simulink model "GS_model"  (R2018b)
settings: Solver=ode5  StartTime=0.0  StopTime=SimuStopTime  FixedStep=T_Simu  RelTol=1e-3
InitFcn:
  | Initial
undefined symbols (not defined in the file or in its folder): Aba10, Aba20, aeroCIP2006_S, aeroCIP2006_X, aeroCIP2006_Y, Agl0, Ass_kS, Ass_n1, Ass_n2, Ass_n3, Ass_n4, Ass_Noise, Ass_R, Ass_Resolution, Ass_TmOrder, AssA_Fix_Abs, AssB_Fix_Abs, AssC_Fix_Abs, AssD_Fix_Abs, AssE_Fix_Aps, AssF_Fix_Aps, C, c_max, c_min, Cd, CenterOfFigNX, CenterOfFigNY, CenterOfFigNZ, CenterOfFigP1, CenterOfFigP2, CenterOfFigPX, CenterOfFigPY, CenterOfFigPZ, Cmu, Crou, DEG2RAD, DiscIntNeverNeededParam, Eg_Dir, Eg_F, Eg_PrepareTime, Eg_r_L_L, Fw_Abf, Fw_Hmax, Fw_J, Fw_Spd0, Fw_Tmax, git_hash_BaseLine, git_hash_Project, Gnss_Noise_Pos, Gnss_Noise_Vel, Gnss_PropgationTime, GyroA_Fix_Abg, GyroA_Noise, GyroB_Fix_Abg, GyroB_Noise, GyroC_Fix_Abg, GyroC_Noise, GyroD_Fix_Abg, GyroD_Noise, h ... (+94)
libraries: simulink x308, sharedutil x46, aerolibutil x37, sharedtransform x31, vrlib x14, aerolibgravity2 x2
(part 11 of 20)

== system GS_model/Subsystem2/Subsystem/Sensor/Ass/BodyAss(A&B&C&D)Model/Subsystem/AssErrModel ==
  AssCur : Inport
  TC_AssGNDSet : Inport  Port=2
  TC_AssErr_Constant : Inport  Port=3
  TC_AssErr_WildValue : Inport  Port=4
  TC_AssErr_Jump : Inport  Port=5
  TC_AssErr_Wave : Inport  Port=6
  AssNum : Inport  Port=7
  AssErrSet : Subsystem
  Constant : Constant  Value=0
  Demux : Demux  Outputs=2
  Demux1 : Demux  Outputs=2
  Demux2 : Demux  Outputs=[1;3]
  Demux3 : Demux  Outputs=[1;2]
  Demux4 : Demux  Outputs=[1;4]
  Demux5 : Demux  Outputs=[1;5]
  If : If  IfExpression=u1 == 1
  If Action Subsystem : Subsystem  TreatAsAtomicUnit=on
  If Action Subsystem1 : Subsystem  TreatAsAtomicUnit=on
  Logical Operator{1..5} (5 alike) : Logic  Operator=OR  AllPortsSameDT=off  OutDataTypeStr=boolean
  Merge : Merge
  Relational Operator{1..10} (10 alike) : RelationalOperator  Operator===  OutDataTypeStr=boolean  RndMeth=Simplest
  Triggered Subsystem1 : Subsystem  TreatAsAtomicUnit=on
      mask Display: disp('AssChoice')
  Triggered Subsystem2 : Subsystem  TreatAsAtomicUnit=on
      mask Display: disp('AssChoice')
  Triggered Subsystem3 : Subsystem  TreatAsAtomicUnit=on
      mask Display: disp('AssChoice')
  Triggered Subsystem4 : Subsystem  TreatAsAtomicUnit=on
      mask Display: disp('AssChoice')
  Triggered Subsystem5 : Subsystem  TreatAsAtomicUnit=on
      mask Display: disp('AssChoice')
  TM_Ass_Cur : Outport
  wires:
  Demux/2 -> Triggered Subsystem1/1(In1)
  Demux/1 -> Relational Operator9/2, Relational Operator2/2
  Demux2/1 -> Relational Operator4/2, Relational Operator7/2
  Demux3/1 -> Relational Operator6/2, Relational Operator5/2
  Demux3/2 -> Triggered Subsystem4/1(In1)
  TC_AssErr_Constant/1 -> Demux/1
  TC_AssErr_Wave/1 -> Demux3/1
  AssCur/1 -> AssErrSet/1(AssCur)
  Triggered Subsystem1/1(Out1) -> AssErrSet/2(TC_AssErr_Constant)
  Triggered Subsystem3/1(Out1) -> AssErrSet/4(TC_AssErr_Jump)
  Triggered Subsystem4/1(Out1) -> AssErrSet/5(TC_StErr_Wave)
  Demux4/1 -> If/1
  If/1 -> If Action Subsystem/Action
  Demux4/2 -> If Action Subsystem/1(In1)
  If/2 -> If Action Subsystem1/Action
  AssErrSet/1(TM_Ass_Cur) -> If Action Subsystem1/1(In1)
  If Action Subsystem/1(Out1) -> Merge/1
  If Action Subsystem1/1(Out1) -> Merge/2
  Merge/1 -> TM_Ass_Cur/1
  Demux2/2 -> Triggered Subsystem3/1(In1)
  TC_AssErr_Jump/1 -> Demux2/1
  TC_AssErr_WildValue/1 -> Demux1/1
  Demux1/1 -> Relational Operator8/2, Relational Operator3/2
  Demux1/2 -> Triggered Subsystem2/1(In1)
  Triggered Subsystem2/1(Out1) -> AssErrSet/3(TC_AssErr_WildValue)
  TC_AssGNDSet/1 -> Demux5/1
  Demux5/1 -> Relational Operator10/2, Relational Operator1/2
  Demux5/2 -> Triggered Subsystem5/1(In1)
  Triggered Subsystem5/1(Out1) -> Demux4/1
  AssNum/1 -> Relational Operator1/1, Relational Operator2/1, Relational Operator3/1, Relational Operator5/1, Relational Operator4/1
  Relational Operator6/1 -> Logical Operator2/1
  Relational Operator5/1 -> Logical Operator2/2
  Logical Operator2/1 -> Triggered Subsystem4/Enable
  Constant/1 -> Relational Operator10/1, Relational Operator9/1, Relational Operator8/1, Relational Operator7/1, Relational Operator6/1
  Relational Operator7/1 -> Logical Operator1/1
  Relational Operator4/1 -> Logical Operator1/2
  Logical Operator1/1 -> Triggered Subsystem3/Enable
  Relational Operator3/1 -> Logical Operator3/2
  Relational Operator8/1 -> Logical Operator3/1
  Logical Operator3/1 -> Triggered Subsystem2/Enable
  Relational Operator9/1 -> Logical Operator4/1
  Relational Operator2/1 -> Logical Operator4/2
  Logical Operator4/1 -> Triggered Subsystem1/Enable
  Relational Operator10/1 -> Logical Operator5/1
  Relational Operator1/1 -> Logical Operator5/2
  Logical Operator5/1 -> Triggered Subsystem5/Enable

== system GS_model/Subsystem2/Subsystem/Sensor/Ass/BodyAss(A&B&C&D)Model/Subsystem/AssMathModel ==
  note: Sun_s
  Sunshine : Inport
  AbAss : Inport  Port=2
  Sun_b : Inport  Port=3
  kS_Ass : Inport  Port=4
  1/ R_Ass : Gain  Gain=1/Ass_R
  A2mA : Gain  Gain=1000
  AssNoise : RandomNumber  Mean=zeros(4,1)  Variance=(Ass_Noise/3)^2*ones(4,1)  Seed=[1:4]  SampleTime=T_Simu
  Compare To Zero{,1..3} (4 alike) : simulink/Logic and Bit Operations/Compare To Zero  relop=>=  OutDataTypeStr=uint8
  Data Type Conversion{,1..3} (4 alike) : DataTypeConversion  OutDataTypeStr=double
  Dot Product{,1..3} (4 alike) : DotProduct  InputSameDT=on  OutDataTypeStr=Inherit: Inherit via internal rule
  Mux5 : Mux
  Product{,1..2,7} (4 alike) : Product  RndMeth=Zero
  Product{3..6} (4 alike) : Product  Inputs=3  RndMeth=Zero
  Product8 : Product  Multiplication=Matrix(*)  RndMeth=Zero
  Rounding Function : Rounding
  Ss1Face1Normal : Constant  Value=Ass_n1
  Ss1Face2Normal : Constant  Value=Ass_n2
  Ss1Face3Normal : Constant  Value=Ass_n3
  Ss1Face4Normal : Constant  Value=Ass_n4
  Sum1 : Sum  Inputs=++|
  Transpose5 : Math  Operator=transpose  SaturateOnIntegerOverflow=on
  decode : Gain  Gain=Ass_Resolution
  encode : Gain  Gain=1/Ass_Resolution
  mA2A : Gain  Gain=0.001
  AssCur : Outport
  wires:
  Ss1Face1Normal/1 -> Dot Product/2
  Product1/1 -> Mux5/2
  Dot Product/1 -> Product3/2, Compare To Zero/1
  Product7/1 -> Mux5/4
  Dot Product3/1 -> Compare To Zero3/1, Product6/2
  Ss1Face3Normal/1 -> Dot Product2/2
  Ss1Face2Normal/1 -> Dot Product1/2
  Product5/1 -> Product2/2
  kS_Ass/1 -> Product3/3, Product4/3, Product6/3, Product5/3
  Dot Product1/1 -> Compare To Zero1/1, Product4/2
  Product2/1 -> Mux5/3
  Product8/1 -> Dot Product/1, Dot Product1/1, Dot Product2/1, Dot Product3/1
  Transpose5/1 -> Product8/1
  Product/1 -> Mux5/1
  Product6/1 -> Product7/2
  Dot Product2/1 -> Product5/2, Compare To Zero2/1
  Compare To Zero2/1 -> Data Type Conversion2/1
  Data Type Conversion1/1 -> Product4/1
  Sunshine/1 -> Product/1, Product1/1, Product2/1, Product7/1
  Product4/1 -> Product1/2
  Product3/1 -> Product/2
  Ss1Face4Normal/1 -> Dot Product3/2
  Compare To Zero3/1 -> Data Type Conversion3/1
  Compare To Zero/1 -> Data Type Conversion/1
  Data Type Conversion3/1 -> Product6/1
  Data Type Conversion2/1 -> Product5/1
  Data Type Conversion/1 -> Product3/1
  Sun_b/1 -> Product8/2
  AbAss/1 -> Transpose5/1
  Compare To Zero1/1 -> Data Type Conversion1/1
  Mux5/1 -> Sum1/2
  AssNoise/1 -> 1/ R_Ass/1
  1/ R_Ass/1 -> Sum1/1
  mA2A/1 -> AssCur/1
  Sum1/1 -> A2mA/1
  encode/1 -> Rounding Function/1
  Rounding Function/1 -> decode/1
  A2mA/1 -> encode/1
  decode/1 -> mA2A/1

== system GS_model/Subsystem2/Subsystem/Sensor/Ass/BodyAss(A&B&C&D)Model/Subsystem1/AssErrModel ==
  AssCur : Inport
  TC_AssGNDSet : Inport  Port=2
  TC_AssErr_Constant : Inport  Port=3
  TC_AssErr_WildValue : Inport  Port=4
  TC_AssErr_Jump : Inport  Port=5
  TC_AssErr_Wave : Inport  Port=6
  AssNum : Inport  Port=7
  AssErrSet : Subsystem
  Constant : Constant  Value=0
  Demux : Demux  Outputs=2
  Demux1 : Demux  Outputs=2
  Demux2 : Demux  Outputs=[1;3]
  Demux3 : Demux  Outputs=[1;2]
  Demux4 : Demux  Outputs=[1;4]
  Demux5 : Demux  Outputs=[1;5]
  If : If  IfExpression=u1 == 1
  If Action Subsystem : Subsystem  TreatAsAtomicUnit=on
  If Action Subsystem1 : Subsystem  TreatAsAtomicUnit=on
  Logical Operator{1..5} (5 alike) : Logic  Operator=OR  AllPortsSameDT=off  OutDataTypeStr=boolean
  Merge : Merge
  Relational Operator{1..10} (10 alike) : RelationalOperator  Operator===  OutDataTypeStr=boolean  RndMeth=Simplest
  Triggered Subsystem1 : Subsystem  TreatAsAtomicUnit=on
      mask Display: disp('AssChoice')
  Triggered Subsystem2 : Subsystem  TreatAsAtomicUnit=on
      mask Display: disp('AssChoice')
  Triggered Subsystem3 : Subsystem  TreatAsAtomicUnit=on
      mask Display: disp('AssChoice')
  Triggered Subsystem4 : Subsystem  TreatAsAtomicUnit=on
      mask Display: disp('AssChoice')
  Triggered Subsystem5 : Subsystem  TreatAsAtomicUnit=on
      mask Display: disp('AssChoice')
  TM_Ass_Cur : Outport
  wires:
  Logical Operator5/1 -> Triggered Subsystem5/Enable
  Relational Operator1/1 -> Logical Operator5/2
  Relational Operator10/1 -> Logical Operator5/1
  Logical Operator4/1 -> Triggered Subsystem1/Enable
  Relational Operator2/1 -> Logical Operator4/2
  Relational Operator9/1 -> Logical Operator4/1
  Logical Operator3/1 -> Triggered Subsystem2/Enable
  Relational Operator8/1 -> Logical Operator3/1
  Relational Operator3/1 -> Logical Operator3/2
  Logical Operator1/1 -> Triggered Subsystem3/Enable
  Relational Operator4/1 -> Logical Operator1/2
  Relational Operator7/1 -> Logical Operator1/1
  Constant/1 -> Relational Operator6/1, Relational Operator7/1, Relational Operator8/1, Relational Operator9/1, Relational Operator10/1
  Logical Operator2/1 -> Triggered Subsystem4/Enable
  Relational Operator5/1 -> Logical Operator2/2
  Relational Operator6/1 -> Logical Operator2/1
  AssNum/1 -> Relational Operator4/1, Relational Operator5/1, Relational Operator3/1, Relational Operator2/1, Relational Operator1/1
  Triggered Subsystem5/1(Out1) -> Demux4/1
  Demux5/2 -> Triggered Subsystem5/1(In1)
  Demux5/1 -> Relational Operator1/2, Relational Operator10/2
  TC_AssGNDSet/1 -> Demux5/1
  Triggered Subsystem2/1(Out1) -> AssErrSet/3(TC_AssErr_WildValue)
  Demux1/2 -> Triggered Subsystem2/1(In1)
  Demux1/1 -> Relational Operator3/2, Relational Operator8/2
  TC_AssErr_WildValue/1 -> Demux1/1
  TC_AssErr_Jump/1 -> Demux2/1
  Demux2/2 -> Triggered Subsystem3/1(In1)
  Merge/1 -> TM_Ass_Cur/1
  If Action Subsystem1/1(Out1) -> Merge/2
  If Action Subsystem/1(Out1) -> Merge/1
  AssErrSet/1(TM_Ass_Cur) -> If Action Subsystem1/1(In1)
  If/2 -> If Action Subsystem1/Action
  Demux4/2 -> If Action Subsystem/1(In1)
  If/1 -> If Action Subsystem/Action
  Demux4/1 -> If/1
  Triggered Subsystem4/1(Out1) -> AssErrSet/5(TC_StErr_Wave)
  Triggered Subsystem3/1(Out1) -> AssErrSet/4(TC_AssErr_Jump)
  Triggered Subsystem1/1(Out1) -> AssErrSet/2(TC_AssErr_Constant)
  AssCur/1 -> AssErrSet/1(AssCur)
  TC_AssErr_Wave/1 -> Demux3/1
  TC_AssErr_Constant/1 -> Demux/1
  Demux3/2 -> Triggered Subsystem4/1(In1)
  Demux3/1 -> Relational Operator5/2, Relational Operator6/2
  Demux2/1 -> Relational Operator7/2, Relational Operator4/2
  Demux/1 -> Relational Operator2/2, Relational Operator9/2
  Demux/2 -> Triggered Subsystem1/1(In1)

== system GS_model/Subsystem2/Subsystem/Sensor/Ass/BodyAss(A&B&C&D)Model/Subsystem1/AssMathModel ==
  note: Sun_s
  Sunshine : Inport
  AbAss : Inport  Port=2
  Sun_b : Inport  Port=3
  kS_Ass : Inport  Port=4
  1/ R_Ass : Gain  Gain=1/Ass_R
  A2mA : Gain  Gain=1000
  AssNoise : RandomNumber  Mean=zeros(4,1)  Variance=(Ass_Noise/3)^2*ones(4,1)  Seed=[1:4]  SampleTime=T_Simu
  Compare To Zero{,1..3} (4 alike) : simulink/Logic and Bit Operations/Compare To Zero  relop=>=  OutDataTypeStr=uint8
  Data Type Conversion{,1..3} (4 alike) : DataTypeConversion  OutDataTypeStr=double
  Dot Product{,1..3} (4 alike) : DotProduct  InputSameDT=on  OutDataTypeStr=Inherit: Inherit via internal rule
  Mux5 : Mux
  Product{,1..2,7} (4 alike) : Product  RndMeth=Zero
  Product{3..6} (4 alike) : Product  Inputs=3  RndMeth=Zero
  Product8 : Product  Multiplication=Matrix(*)  RndMeth=Zero
  Rounding Function : Rounding
  Ss1Face1Normal : Constant  Value=Ass_n1
  Ss1Face2Normal : Constant  Value=Ass_n2
  Ss1Face3Normal : Constant  Value=Ass_n3
  Ss1Face4Normal : Constant  Value=Ass_n4
  Sum1 : Sum  Inputs=++|
  Transpose5 : Math  Operator=transpose  SaturateOnIntegerOverflow=on
  decode : Gain  Gain=Ass_Resolution
  encode : Gain  Gain=1/Ass_Resolution
  mA2A : Gain  Gain=0.001
  AssCur : Outport
  wires:
  decode/1 -> mA2A/1
  A2mA/1 -> encode/1
  Rounding Function/1 -> decode/1
  encode/1 -> Rounding Function/1
  Sum1/1 -> A2mA/1
  mA2A/1 -> AssCur/1
  1/ R_Ass/1 -> Sum1/1
  AssNoise/1 -> 1/ R_Ass/1
  Mux5/1 -> Sum1/2
  Compare To Zero1/1 -> Data Type Conversion1/1
  AbAss/1 -> Transpose5/1
  Sun_b/1 -> Product8/2
  Data Type Conversion/1 -> Product3/1
  Data Type Conversion2/1 -> Product5/1
  Data Type Conversion3/1 -> Product6/1
  Compare To Zero/1 -> Data Type Conversion/1
  Compare To Zero3/1 -> Data Type Conversion3/1
  Ss1Face4Normal/1 -> Dot Product3/2
  Product3/1 -> Product/2
  Product4/1 -> Product1/2
  Sunshine/1 -> Product7/1, Product2/1, Product1/1, Product/1
  Data Type Conversion1/1 -> Product4/1
  Compare To Zero2/1 -> Data Type Conversion2/1
  Dot Product2/1 -> Compare To Zero2/1, Product5/2
  Product6/1 -> Product7/2
  Product/1 -> Mux5/1
  Transpose5/1 -> Product8/1
  Product8/1 -> Dot Product3/1, Dot Product2/1, Dot Product1/1, Dot Product/1
  Product2/1 -> Mux5/3
  Dot Product1/1 -> Product4/2, Compare To Zero1/1
  kS_Ass/1 -> Product5/3, Product6/3, Product4/3, Product3/3
  Product5/1 -> Product2/2
  Ss1Face2Normal/1 -> Dot Product1/2
  Ss1Face3Normal/1 -> Dot Product2/2
  Dot Product3/1 -> Product6/2, Compare To Zero3/1
  Product7/1 -> Mux5/4
  Dot Product/1 -> Compare To Zero/1, Product3/2
  Product1/1 -> Mux5/2
  Ss1Face1Normal/1 -> Dot Product/2

== system GS_model/Subsystem2/Subsystem/Sensor/Ass/BodyAss(A&B&C&D)Model/Subsystem2/AssErrModel ==
  AssCur : Inport
  TC_AssGNDSet : Inport  Port=2
  TC_AssErr_Constant : Inport  Port=3
  TC_AssErr_WildValue : Inport  Port=4
  TC_AssErr_Jump : Inport  Port=5
  TC_AssErr_Wave : Inport  Port=6
  AssNum : Inport  Port=7
  AssErrSet : Subsystem
  Constant : Constant  Value=0
  Demux : Demux  Outputs=2
  Demux1 : Demux  Outputs=2
  Demux2 : Demux  Outputs=[1;3]
  Demux3 : Demux  Outputs=[1;2]
  Demux4 : Demux  Outputs=[1;4]
  Demux5 : Demux  Outputs=[1;5]
  If : If  IfExpression=u1 == 1
  If Action Subsystem : Subsystem  TreatAsAtomicUnit=on
  If Action Subsystem1 : Subsystem  TreatAsAtomicUnit=on
  Logical Operator{1..5} (5 alike) : Logic  Operator=OR  AllPortsSameDT=off  OutDataTypeStr=boolean
  Merge : Merge
  Relational Operator{1..10} (10 alike) : RelationalOperator  Operator===  OutDataTypeStr=boolean  RndMeth=Simplest
  Triggered Subsystem1 : Subsystem  TreatAsAtomicUnit=on
      mask Display: disp('AssChoice')
  Triggered Subsystem2 : Subsystem  TreatAsAtomicUnit=on
      mask Display: disp('AssChoice')
  Triggered Subsystem3 : Subsystem  TreatAsAtomicUnit=on
      mask Display: disp('AssChoice')
  Triggered Subsystem4 : Subsystem  TreatAsAtomicUnit=on
      mask Display: disp('AssChoice')
  Triggered Subsystem5 : Subsystem  TreatAsAtomicUnit=on
      mask Display: disp('AssChoice')
  TM_Ass_Cur : Outport
  wires:
  Demux/2 -> Triggered Subsystem1/1(In1)
  Demux/1 -> Relational Operator9/2, Relational Operator2/2
  Demux2/1 -> Relational Operator4/2, Relational Operator7/2
  Demux3/1 -> Relational Operator6/2, Relational Operator5/2
  Demux3/2 -> Triggered Subsystem4/1(In1)
  TC_AssErr_Constant/1 -> Demux/1
  TC_AssErr_Wave/1 -> Demux3/1
  AssCur/1 -> AssErrSet/1(AssCur)
  Triggered Subsystem1/1(Out1) -> AssErrSet/2(TC_AssErr_Constant)
  Triggered Subsystem3/1(Out1) -> AssErrSet/4(TC_AssErr_Jump)
  Triggered Subsystem4/1(Out1) -> AssErrSet/5(TC_StErr_Wave)
  Demux4/1 -> If/1
  If/1 -> If Action Subsystem/Action
  Demux4/2 -> If Action Subsystem/1(In1)
  If/2 -> If Action Subsystem1/Action
  AssErrSet/1(TM_Ass_Cur) -> If Action Subsystem1/1(In1)
  If Action Subsystem/1(Out1) -> Merge/1
  If Action Subsystem1/1(Out1) -> Merge/2
  Merge/1 -> TM_Ass_Cur/1
  Demux2/2 -> Triggered Subsystem3/1(In1)
  TC_AssErr_Jump/1 -> Demux2/1
  TC_AssErr_WildValue/1 -> Demux1/1
  Demux1/1 -> Relational Operator8/2, Relational Operator3/2
  Demux1/2 -> Triggered Subsystem2/1(In1)
  Triggered Subsystem2/1(Out1) -> AssErrSet/3(TC_AssErr_WildValue)
  TC_AssGNDSet/1 -> Demux5/1
  Demux5/1 -> Relational Operator10/2, Relational Operator1/2
  Demux5/2 -> Triggered Subsystem5/1(In1)
  Triggered Subsystem5/1(Out1) -> Demux4/1
  AssNum/1 -> Relational Operator1/1, Relational Operator2/1, Relational Operator3/1, Relational Operator5/1, Relational Operator4/1
  Relational Operator6/1 -> Logical Operator2/1
  Relational Operator5/1 -> Logical Operator2/2
  Logical Operator2/1 -> Triggered Subsystem4/Enable
  Constant/1 -> Relational Operator10/1, Relational Operator9/1, Relational Operator8/1, Relational Operator7/1, Relational Operator6/1
  Relational Operator7/1 -> Logical Operator1/1
  Relational Operator4/1 -> Logical Operator1/2
  Logical Operator1/1 -> Triggered Subsystem3/Enable
  Relational Operator3/1 -> Logical Operator3/2
  Relational Operator8/1 -> Logical Operator3/1
  Logical Operator3/1 -> Triggered Subsystem2/Enable
  Relational Operator9/1 -> Logical Operator4/1
  Relational Operator2/1 -> Logical Operator4/2
  Logical Operator4/1 -> Triggered Subsystem1/Enable
  Relational Operator10/1 -> Logical Operator5/1
  Relational Operator1/1 -> Logical Operator5/2
  Logical Operator5/1 -> Triggered Subsystem5/Enable

== system GS_model/Subsystem2/Subsystem/Sensor/Ass/BodyAss(A&B&C&D)Model/Subsystem2/AssMathModel ==
  note: Sun_s
  Sunshine : Inport
  AbAss : Inport  Port=2
  Sun_b : Inport  Port=3
  kS_Ass : Inport  Port=4
  1/ R_Ass : Gain  Gain=1/Ass_R
  A2mA : Gain  Gain=1000
  AssNoise : RandomNumber  Mean=zeros(4,1)  Variance=(Ass_Noise/3)^2*ones(4,1)  Seed=[1:4]  SampleTime=T_Simu
  Compare To Zero{,1..3} (4 alike) : simulink/Logic and Bit Operations/Compare To Zero  relop=>=  OutDataTypeStr=uint8
  Data Type Conversion{,1..3} (4 alike) : DataTypeConversion  OutDataTypeStr=double
  Dot Product{,1..3} (4 alike) : DotProduct  InputSameDT=on  OutDataTypeStr=Inherit: Inherit via internal rule
  Mux5 : Mux
  Product{,1..2,7} (4 alike) : Product  RndMeth=Zero
  Product{3..6} (4 alike) : Product  Inputs=3  RndMeth=Zero
  Product8 : Product  Multiplication=Matrix(*)  RndMeth=Zero
  Rounding Function : Rounding
  Ss1Face1Normal : Constant  Value=Ass_n1
  Ss1Face2Normal : Constant  Value=Ass_n2
  Ss1Face3Normal : Constant  Value=Ass_n3
  Ss1Face4Normal : Constant  Value=Ass_n4
  Sum1 : Sum  Inputs=++|
  Transpose5 : Math  Operator=transpose  SaturateOnIntegerOverflow=on
  decode : Gain  Gain=Ass_Resolution
  encode : Gain  Gain=1/Ass_Resolution
  mA2A : Gain  Gain=0.001
  AssCur : Outport
  wires:
  Ss1Face1Normal/1 -> Dot Product/2
  Product1/1 -> Mux5/2
  Dot Product/1 -> Product3/2, Compare To Zero/1
  Product7/1 -> Mux5/4
  Dot Product3/1 -> Compare To Zero3/1, Product6/2
  Ss1Face3Normal/1 -> Dot Product2/2
  Ss1Face2Normal/1 -> Dot Product1/2
  Product5/1 -> Product2/2
  kS_Ass/1 -> Product3/3, Product4/3, Product6/3, Product5/3
  Dot Product1/1 -> Compare To Zero1/1, Product4/2
  Product2/1 -> Mux5/3
  Product8/1 -> Dot Product/1, Dot Product1/1, Dot Product2/1, Dot Product3/1
  Transpose5/1 -> Product8/1
  Product/1 -> Mux5/1
  Product6/1 -> Product7/2
  Dot Product2/1 -> Product5/2, Compare To Zero2/1
  Compare To Zero2/1 -> Data Type Conversion2/1
  Data Type Conversion1/1 -> Product4/1
  Sunshine/1 -> Product/1, Product1/1, Product2/1, Product7/1
  Product4/1 -> Product1/2
  Product3/1 -> Product/2
  Ss1Face4Normal/1 -> Dot Product3/2
  Compare To Zero3/1 -> Data Type Conversion3/1
  Compare To Zero/1 -> Data Type Conversion/1
  Data Type Conversion3/1 -> Product6/1
  Data Type Conversion2/1 -> Product5/1
  Data Type Conversion/1 -> Product3/1
  Sun_b/1 -> Product8/2
  AbAss/1 -> Transpose5/1
  Compare To Zero1/1 -> Data Type Conversion1/1
  Mux5/1 -> Sum1/2
  AssNoise/1 -> 1/ R_Ass/1
  1/ R_Ass/1 -> Sum1/1
  mA2A/1 -> AssCur/1
  Sum1/1 -> A2mA/1
  encode/1 -> Rounding Function/1
  Rounding Function/1 -> decode/1
  A2mA/1 -> encode/1
  decode/1 -> mA2A/1

== system GS_model/Subsystem2/Subsystem/Sensor/Ass/BodyAss(A&B&C&D)Model/Subsystem3/AssErrModel ==
  AssCur : Inport
  TC_AssGNDSet : Inport  Port=2
  TC_AssErr_Constant : Inport  Port=3
  TC_AssErr_WildValue : Inport  Port=4
  TC_AssErr_Jump : Inport  Port=5
  TC_AssErr_Wave : Inport  Port=6
  AssNum : Inport  Port=7
  AssErrSet : Subsystem
  Constant : Constant  Value=0
  Demux : Demux  Outputs=2
  Demux1 : Demux  Outputs=2
  Demux2 : Demux  Outputs=[1;3]
  Demux3 : Demux  Outputs=[1;2]
  Demux4 : Demux  Outputs=[1;4]
  Demux5 : Demux  Outputs=[1;5]
  If : If  IfExpression=u1 == 1
  If Action Subsystem : Subsystem  TreatAsAtomicUnit=on
  If Action Subsystem1 : Subsystem  TreatAsAtomicUnit=on
  Logical Operator{1..5} (5 alike) : Logic  Operator=OR  AllPortsSameDT=off  OutDataTypeStr=boolean
  Merge : Merge
  Relational Operator{1..10} (10 alike) : RelationalOperator  Operator===  OutDataTypeStr=boolean  RndMeth=Simplest
  Triggered Subsystem1 : Subsystem  TreatAsAtomicUnit=on
      mask Display: disp('AssChoice')
  Triggered Subsystem2 : Subsystem  TreatAsAtomicUnit=on
      mask Display: disp('AssChoice')
  Triggered Subsystem3 : Subsystem  TreatAsAtomicUnit=on
      mask Display: disp('AssChoice')
  Triggered Subsystem4 : Subsystem  TreatAsAtomicUnit=on
      mask Display: disp('AssChoice')
  Triggered Subsystem5 : Subsystem  TreatAsAtomicUnit=on
      mask Display: disp('AssChoice')
  TM_Ass_Cur : Outport
  wires:
  Logical Operator5/1 -> Triggered Subsystem5/Enable
  Relational Operator1/1 -> Logical Operator5/2
  Relational Operator10/1 -> Logical Operator5/1
  Logical Operator4/1 -> Triggered Subsystem1/Enable
  Relational Operator2/1 -> Logical Operator4/2
  Relational Operator9/1 -> Logical Operator4/1
  Logical Operator3/1 -> Triggered Subsystem2/Enable
  Relational Operator8/1 -> Logical Operator3/1
  Relational Operator3/1 -> Logical Operator3/2
  Logical Operator1/1 -> Triggered Subsystem3/Enable
  Relational Operator4/1 -> Logical Operator1/2
  Relational Operator7/1 -> Logical Operator1/1
  Constant/1 -> Relational Operator6/1, Relational Operator7/1, Relational Operator8/1, Relational Operator9/1, Relational Operator10/1
  Logical Operator2/1 -> Triggered Subsystem4/Enable
  Relational Operator5/1 -> Logical Operator2/2
  Relational Operator6/1 -> Logical Operator2/1
  AssNum/1 -> Relational Operator4/1, Relational Operator5/1, Relational Operator3/1, Relational Operator2/1, Relational Operator1/1
  Triggered Subsystem5/1(Out1) -> Demux4/1
  Demux5/2 -> Triggered Subsystem5/1(In1)
  Demux5/1 -> Relational Operator1/2, Relational Operator10/2
  TC_AssGNDSet/1 -> Demux5/1
  Triggered Subsystem2/1(Out1) -> AssErrSet/3(TC_AssErr_WildValue)
  Demux1/2 -> Triggered Subsystem2/1(In1)
  Demux1/1 -> Relational Operator3/2, Relational Operator8/2
  TC_AssErr_WildValue/1 -> Demux1/1
  TC_AssErr_Jump/1 -> Demux2/1
  Demux2/2 -> Triggered Subsystem3/1(In1)
  Merge/1 -> TM_Ass_Cur/1
  If Action Subsystem1/1(Out1) -> Merge/2
  If Action Subsystem/1(Out1) -> Merge/1
  AssErrSet/1(TM_Ass_Cur) -> If Action Subsystem1/1(In1)
  If/2 -> If Action Subsystem1/Action
  Demux4/2 -> If Action Subsystem/1(In1)
  If/1 -> If Action Subsystem/Action
  Demux4/1 -> If/1
  Triggered Subsystem4/1(Out1) -> AssErrSet/5(TC_StErr_Wave)
  Triggered Subsystem3/1(Out1) -> AssErrSet/4(TC_AssErr_Jump)
  Triggered Subsystem1/1(Out1) -> AssErrSet/2(TC_AssErr_Constant)
  AssCur/1 -> AssErrSet/1(AssCur)
  TC_AssErr_Wave/1 -> Demux3/1
  TC_AssErr_Constant/1 -> Demux/1
  Demux3/2 -> Triggered Subsystem4/1(In1)
  Demux3/1 -> Relational Operator5/2, Relational Operator6/2
  Demux2/1 -> Relational Operator7/2, Relational Operator4/2
  Demux/1 -> Relational Operator2/2, Relational Operator9/2
  Demux/2 -> Triggered Subsystem1/1(In1)

== system GS_model/Subsystem2/Subsystem/Sensor/Ass/BodyAss(A&B&C&D)Model/Subsystem3/AssMathModel ==
  note: Sun_s
  Sunshine : Inport
  AbAss : Inport  Port=2
  Sun_b : Inport  Port=3
  kS_Ass : Inport  Port=4
  1/ R_Ass : Gain  Gain=1/Ass_R
  A2mA : Gain  Gain=1000
  AssNoise : RandomNumber  Mean=zeros(4,1)  Variance=(Ass_Noise/3)^2*ones(4,1)  Seed=[1:4]  SampleTime=T_Simu
  Compare To Zero{,1..3} (4 alike) : simulink/Logic and Bit Operations/Compare To Zero  relop=>=  OutDataTypeStr=uint8
  Data Type Conversion{,1..3} (4 alike) : DataTypeConversion  OutDataTypeStr=double
  Dot Product{,1..3} (4 alike) : DotProduct  InputSameDT=on  OutDataTypeStr=Inherit: Inherit via internal rule
  Mux5 : Mux
  Product{,1..2,7} (4 alike) : Product  RndMeth=Zero
  Product{3..6} (4 alike) : Product  Inputs=3  RndMeth=Zero
  Product8 : Product  Multiplication=Matrix(*)  RndMeth=Zero
  Rounding Function : Rounding
  Ss1Face1Normal : Constant  Value=Ass_n1
  Ss1Face2Normal : Constant  Value=Ass_n2
  Ss1Face3Normal : Constant  Value=Ass_n3
  Ss1Face4Normal : Constant  Value=Ass_n4
  Sum1 : Sum  Inputs=++|
  Transpose5 : Math  Operator=transpose  SaturateOnIntegerOverflow=on
  decode : Gain  Gain=Ass_Resolution
  encode : Gain  Gain=1/Ass_Resolution
  mA2A : Gain  Gain=0.001
  AssCur : Outport
  wires:
  decode/1 -> mA2A/1
  A2mA/1 -> encode/1
  Rounding Function/1 -> decode/1
  encode/1 -> Rounding Function/1
  Sum1/1 -> A2mA/1
  mA2A/1 -> AssCur/1
  1/ R_Ass/1 -> Sum1/1
  AssNoise/1 -> 1/ R_Ass/1
  Mux5/1 -> Sum1/2
  Compare To Zero1/1 -> Data Type Conversion1/1
  AbAss/1 -> Transpose5/1
  Sun_b/1 -> Product8/2
  Data Type Conversion/1 -> Product3/1
  Data Type Conversion2/1 -> Product5/1
  Data Type Conversion3/1 -> Product6/1
  Compare To Zero/1 -> Data Type Conversion/1
  Compare To Zero3/1 -> Data Type Conversion3/1
  Ss1Face4Normal/1 -> Dot Product3/2
  Product3/1 -> Product/2
  Product4/1 -> Product1/2
  Sunshine/1 -> Product7/1, Product2/1, Product1/1, Product/1
  Data Type Conversion1/1 -> Product4/1
  Compare To Zero2/1 -> Data Type Conversion2/1
  Dot Product2/1 -> Compare To Zero2/1, Product5/2
  Product6/1 -> Product7/2
  Product/1 -> Mux5/1
  Transpose5/1 -> Product8/1
  Product8/1 -> Dot Product3/1, Dot Product2/1, Dot Product1/1, Dot Product/1
  Product2/1 -> Mux5/3
  Dot Product1/1 -> Product4/2, Compare To Zero1/1
  kS_Ass/1 -> Product5/3, Product6/3, Product4/3, Product3/3
  Product5/1 -> Product2/2
  Ss1Face2Normal/1 -> Dot Product1/2
  Ss1Face3Normal/1 -> Dot Product2/2
  Dot Product3/1 -> Product6/2, Compare To Zero3/1
  Product7/1 -> Mux5/4
  Dot Product/1 -> Compare To Zero/1, Product3/2
  Product1/1 -> Mux5/2
  Ss1Face1Normal/1 -> Dot Product/2

== system GS_model/Subsystem2/Subsystem/Sensor/Ass/SolarPanelAss(E&F)Model/Subsystem/AssErrModel ==
  AssCur : Inport
  TC_AssGNDSet : Inport  Port=2
  TC_AssErr_Constant : Inport  Port=3
  TC_AssErr_WildValue : Inport  Port=4
  TC_AssErr_Jump : Inport  Port=5
  TC_AssErr_Wave : Inport  Port=6
  AssNum : Inport  Port=7
  AssErrSet : Subsystem
  Constant : Constant  Value=0
  Demux : Demux  Outputs=2
  Demux1 : Demux  Outputs=2
  Demux2 : Demux  Outputs=[1;3]
  Demux3 : Demux  Outputs=[1;2]
  Demux4 : Demux  Outputs=[1;4]
  Demux5 : Demux  Outputs=[1;5]
  If : If  IfExpression=u1 == 1
  If Action Subsystem : Subsystem  TreatAsAtomicUnit=on
  If Action Subsystem1 : Subsystem  TreatAsAtomicUnit=on
  Logical Operator{1..5} (5 alike) : Logic  Operator=OR  AllPortsSameDT=off  OutDataTypeStr=boolean
  Merge : Merge
  Relational Operator{1..10} (10 alike) : RelationalOperator  Operator===  OutDataTypeStr=boolean  RndMeth=Simplest
  Triggered Subsystem1 : Subsystem  TreatAsAtomicUnit=on
      mask Display: disp('AssChoice')
  Triggered Subsystem2 : Subsystem  TreatAsAtomicUnit=on
      mask Display: disp('AssChoice')
  Triggered Subsystem3 : Subsystem  TreatAsAtomicUnit=on
      mask Display: disp('AssChoice')
  Triggered Subsystem4 : Subsystem  TreatAsAtomicUnit=on
      mask Display: disp('AssChoice')
  Triggered Subsystem5 : Subsystem  TreatAsAtomicUnit=on
      mask Display: disp('AssChoice')
  TM_Ass_Cur : Outport
  wires:
  Demux/2 -> Triggered Subsystem1/1(In1)
  Demux/1 -> Relational Operator9/2, Relational Operator2/2
  Demux2/1 -> Relational Operator4/2, Relational Operator7/2
  Demux3/1 -> Relational Operator6/2, Relational Operator5/2
  Demux3/2 -> Triggered Subsystem4/1(In1)
  TC_AssErr_Constant/1 -> Demux/1
  TC_AssErr_Wave/1 -> Demux3/1
  AssCur/1 -> AssErrSet/1(AssCur)
  Triggered Subsystem1/1(Out1) -> AssErrSet/2(TC_AssErr_Constant)
  Triggered Subsystem3/1(Out1) -> AssErrSet/4(TC_AssErr_Jump)
  Triggered Subsystem4/1(Out1) -> AssErrSet/5(TC_StErr_Wave)
  Demux4/1 -> If/1
  If/1 -> If Action Subsystem/Action
  Demux4/2 -> If Action Subsystem/1(In1)
  If/2 -> If Action Subsystem1/Action
  AssErrSet/1(TM_Ass_Cur) -> If Action Subsystem1/1(In1)
  If Action Subsystem/1(Out1) -> Merge/1
  If Action Subsystem1/1(Out1) -> Merge/2
  Merge/1 -> TM_Ass_Cur/1
  Demux2/2 -> Triggered Subsystem3/1(In1)
  TC_AssErr_Jump/1 -> Demux2/1
  TC_AssErr_WildValue/1 -> Demux1/1
  Demux1/1 -> Relational Operator8/2, Relational Operator3/2
  Demux1/2 -> Triggered Subsystem2/1(In1)
  Triggered Subsystem2/1(Out1) -> AssErrSet/3(TC_AssErr_WildValue)
  TC_AssGNDSet/1 -> Demux5/1
  Demux5/1 -> Relational Operator10/2, Relational Operator1/2
  Demux5/2 -> Triggered Subsystem5/1(In1)
  Triggered Subsystem5/1(Out1) -> Demux4/1
  AssNum/1 -> Relational Operator1/1, Relational Operator2/1, Relational Operator3/1, Relational Operator5/1, Relational Operator4/1
  Relational Operator6/1 -> Logical Operator2/1
  Relational Operator5/1 -> Logical Operator2/2
  Logical Operator2/1 -> Triggered Subsystem4/Enable
  Constant/1 -> Relational Operator10/1, Relational Operator9/1, Relational Operator8/1, Relational Operator7/1, Relational Operator6/1
  Relational Operator7/1 -> Logical Operator1/1
  Relational Operator4/1 -> Logical Operator1/2
  Logical Operator1/1 -> Triggered Subsystem3/Enable
  Relational Operator3/1 -> Logical Operator3/2
  Relational Operator8/1 -> Logical Operator3/1
  Logical Operator3/1 -> Triggered Subsystem2/Enable
  Relational Operator9/1 -> Logical Operator4/1
  Relational Operator2/1 -> Logical Operator4/2
  Logical Operator4/1 -> Triggered Subsystem1/Enable
  Relational Operator10/1 -> Logical Operator5/1
  Relational Operator1/1 -> Logical Operator5/2
  Logical Operator5/1 -> Triggered Subsystem5/Enable

== system GS_model/Subsystem2/Subsystem/Sensor/Ass/SolarPanelAss(E&F)Model/Subsystem/AssMathModel ==
  note: A
  note: Sun_s
  Sunshine : Inport
  ApAss : Inport  Port=2
  Sun_b : Inport  Port=3
  kS_Ass : Inport  Port=4
  Abp_PY : Inport  Port=5
  1/ R_Ass : Gain  Gain=1/Ass_R
  A2mA : Gain  Gain=1000
  AssNoise : RandomNumber  Mean=zeros(4,1)  Variance=(Ass_Noise/3)^2*ones(4,1)  Seed=[5:8]  SampleTime=T_Simu
  Compare To Zero{,1..3} (4 alike) : simulink/Logic and Bit Operations/Compare To Zero  relop=>=  OutDataTypeStr=uint8
  Data Type Conversion{,1..3} (4 alike) : DataTypeConversion  OutDataTypeStr=double
  Dot Product{,1..3} (4 alike) : DotProduct  InputSameDT=on  OutDataTypeStr=Inherit: Inherit via internal rule
  Mux5 : Mux
  Product{,1..2,7} (4 alike) : Product  RndMeth=Zero
  Product{3..6} (4 alike) : Product  Inputs=3  RndMeth=Zero
  Product8 : Product  Multiplication=Matrix(*)  RndMeth=Zero
  Product9 : Product  Multiplication=Matrix(*)  RndMeth=Zero
  Rounding Function : Rounding
  Ss1Face1Normal : Constant  Value=Ass_n1
  Ss1Face2Normal : Constant  Value=Ass_n2
  Ss1Face3Normal : Constant  Value=Ass_n3
  Ss1Face4Normal : Constant  Value=Ass_n4
  Sum1 : Sum  Inputs=++|
  Transpose5 : Math  Operator=transpose  SaturateOnIntegerOverflow=on
  decode : Gain  Gain=Ass_Resolution
  encode : Gain  Gain=1/Ass_Resolution
  mA2A : Gain  Gain=0.001
  AssCur : Outport
  wires:
  decode/1 -> mA2A/1
  A2mA/1 -> encode/1
  Rounding Function/1 -> decode/1
  encode/1 -> Rounding Function/1
  Sum1/1 -> A2mA/1
  mA2A/1 -> AssCur/1
  1/ R_Ass/1 -> Sum1/1
  AssNoise/1 -> 1/ R_Ass/1
  Mux5/1 -> Sum1/2
  Compare To Zero1/1 -> Data Type Conversion1/1
  Sun_b/1 -> Product8/2
  Data Type Conversion/1 -> Product3/1
  Data Type Conversion2/1 -> Product5/1
  Data Type Conversion3/1 -> Product6/1
  Compare To Zero/1 -> Data Type Conversion/1
  Compare To Zero3/1 -> Data Type Conversion3/1
  Ss1Face4Normal/1 -> Dot Product3/2
  Product3/1 -> Product/2
  Product4/1 -> Product1/2
  Sunshine/1 -> Product7/1, Product2/1, Product1/1, Product/1
  Data Type Conversion1/1 -> Product4/1
  Compare To Zero2/1 -> Data Type Conversion2/1
  Dot Product2/1 -> Compare To Zero2/1, Product5/2
  Product6/1 -> Product7/2
  Product/1 -> Mux5/1
  Transpose5/1 -> Product8/1
  Product8/1 -> Dot Product3/1, Dot Product2/1, Dot Product1/1, Dot Product/1
  Product2/1 -> Mux5/3
  Dot Product1/1 -> Product4/2, Compare To Zero1/1
  kS_Ass/1 -> Product5/3, Product6/3, Product4/3, Product3/3
  Product5/1 -> Product2/2
  Ss1Face2Normal/1 -> Dot Product1/2
  Ss1Face3Normal/1 -> Dot Product2/2
  Dot Product3/1 -> Product6/2, Compare To Zero3/1
  Product7/1 -> Mux5/4
  Dot Product/1 -> Compare To Zero/1, Product3/2
  Product1/1 -> Mux5/2
  Ss1Face1Normal/1 -> Dot Product/2
  Abp_PY/1 -> Product9/1
  ApAss/1 -> Product9/2
  Product9/1 -> Transpose5/1

== system GS_model/Subsystem2/Subsystem/Sensor/Ass/SolarPanelAss(E&F)Model/Subsystem1/AssErrModel ==
  AssCur : Inport
  TC_AssGNDSet : Inport  Port=2
  TC_AssErr_Constant : Inport  Port=3
  TC_AssErr_WildValue : Inport  Port=4
  TC_AssErr_Jump : Inport  Port=5
  TC_AssErr_Wave : Inport  Port=6
  AssNum : Inport  Port=7
  AssErrSet : Subsystem
  Constant : Constant  Value=0
  Demux : Demux  Outputs=2
  Demux1 : Demux  Outputs=2
  Demux2 : Demux  Outputs=[1;3]
  Demux3 : Demux  Outputs=[1;2]
  Demux4 : Demux  Outputs=[1;4]
  Demux5 : Demux  Outputs=[1;5]
  If : If  IfExpression=u1 == 1
  If Action Subsystem : Subsystem  TreatAsAtomicUnit=on
  If Action Subsystem1 : Subsystem  TreatAsAtomicUnit=on
  Logical Operator{1..5} (5 alike) : Logic  Operator=OR  AllPortsSameDT=off  OutDataTypeStr=boolean
  Merge : Merge
  Relational Operator{1..10} (10 alike) : RelationalOperator  Operator===  OutDataTypeStr=boolean  RndMeth=Simplest
  Triggered Subsystem1 : Subsystem  TreatAsAtomicUnit=on
      mask Display: disp('AssChoice')
  Triggered Subsystem2 : Subsystem  TreatAsAtomicUnit=on
      mask Display: disp('AssChoice')
  Triggered Subsystem3 : Subsystem  TreatAsAtomicUnit=on
      mask Display: disp('AssChoice')
  Triggered Subsystem4 : Subsystem  TreatAsAtomicUnit=on
      mask Display: disp('AssChoice')
  Triggered Subsystem5 : Subsystem  TreatAsAtomicUnit=on
      mask Display: disp('AssChoice')
  TM_Ass_Cur : Outport
  wires:
  Demux/2 -> Triggered Subsystem1/1(In1)
  Demux/1 -> Relational Operator9/2, Relational Operator2/2
  Demux2/1 -> Relational Operator4/2, Relational Operator7/2
  Demux3/1 -> Relational Operator6/2, Relational Operator5/2
  Demux3/2 -> Triggered Subsystem4/1(In1)
  TC_AssErr_Constant/1 -> Demux/1
  TC_AssErr_Wave/1 -> Demux3/1
  AssCur/1 -> AssErrSet/1(AssCur)
  Triggered Subsystem1/1(Out1) -> AssErrSet/2(TC_AssErr_Constant)
  Triggered Subsystem3/1(Out1) -> AssErrSet/4(TC_AssErr_Jump)
  Triggered Subsystem4/1(Out1) -> AssErrSet/5(TC_StErr_Wave)
  Demux4/1 -> If/1
  If/1 -> If Action Subsystem/Action
  Demux4/2 -> If Action Subsystem/1(In1)
  If/2 -> If Action Subsystem1/Action
  AssErrSet/1(TM_Ass_Cur) -> If Action Subsystem1/1(In1)
  If Action Subsystem/1(Out1) -> Merge/1
  If Action Subsystem1/1(Out1) -> Merge/2
  Merge/1 -> TM_Ass_Cur/1
  Demux2/2 -> Triggered Subsystem3/1(In1)
  TC_AssErr_Jump/1 -> Demux2/1
  TC_AssErr_WildValue/1 -> Demux1/1
  Demux1/1 -> Relational Operator8/2, Relational Operator3/2
  Demux1/2 -> Triggered Subsystem2/1(In1)
  Triggered Subsystem2/1(Out1) -> AssErrSet/3(TC_AssErr_WildValue)
  TC_AssGNDSet/1 -> Demux5/1
  Demux5/1 -> Relational Operator10/2, Relational Operator1/2
  Demux5/2 -> Triggered Subsystem5/1(In1)
  Triggered Subsystem5/1(Out1) -> Demux4/1
  AssNum/1 -> Relational Operator1/1, Relational Operator2/1, Relational Operator3/1, Relational Operator5/1, Relational Operator4/1
  Relational Operator6/1 -> Logical Operator2/1
  Relational Operator5/1 -> Logical Operator2/2
  Logical Operator2/1 -> Triggered Subsystem4/Enable
  Constant/1 -> Relational Operator10/1, Relational Operator9/1, Relational Operator8/1, Relational Operator7/1, Relational Operator6/1
  Relational Operator7/1 -> Logical Operator1/1
  Relational Operator4/1 -> Logical Operator1/2
  Logical Operator1/1 -> Triggered Subsystem3/Enable
  Relational Operator3/1 -> Logical Operator3/2
  Relational Operator8/1 -> Logical Operator3/1
  Logical Operator3/1 -> Triggered Subsystem2/Enable
  Relational Operator9/1 -> Logical Operator4/1
  Relational Operator2/1 -> Logical Operator4/2
  Logical Operator4/1 -> Triggered Subsystem1/Enable
  Relational Operator10/1 -> Logical Operator5/1
  Relational Operator1/1 -> Logical Operator5/2
  Logical Operator5/1 -> Triggered Subsystem5/Enable

== system GS_model/Subsystem2/Subsystem/Sensor/Ass/SolarPanelAss(E&F)Model/Subsystem1/AssMathModel ==
  note: Sun_s
  note: A
  Sunshine : Inport
  ApAss : Inport  Port=2
  Sun_b : Inport  Port=3
  kS_Ass : Inport  Port=4
  Abp_PY : Inport  Port=5
  1/ R_Ass : Gain  Gain=1/Ass_R
  A2mA : Gain  Gain=1000
  AssNoise : RandomNumber  Mean=zeros(4,1)  Variance=(Ass_Noise/3)^2*ones(4,1)  Seed=[6:9]  SampleTime=T_Simu
  Compare To Zero{,1..3} (4 alike) : simulink/Logic and Bit Operations/Compare To Zero  relop=>=  OutDataTypeStr=uint8
  Data Type Conversion{,1..3} (4 alike) : DataTypeConversion  OutDataTypeStr=double
  Dot Product{,1..3} (4 alike) : DotProduct  InputSameDT=on  OutDataTypeStr=Inherit: Inherit via internal rule
  Mux5 : Mux
  Product{,1..2,7} (4 alike) : Product  RndMeth=Zero
  Product{3..6} (4 alike) : Product  Inputs=3  RndMeth=Zero
  Product8 : Product  Multiplication=Matrix(*)  RndMeth=Zero
  Product9 : Product  Multiplication=Matrix(*)  RndMeth=Zero
  Rounding Function : Rounding
  Ss1Face1Normal : Constant  Value=Ass_n1
  Ss1Face2Normal : Constant  Value=Ass_n2
  Ss1Face3Normal : Constant  Value=Ass_n3
  Ss1Face4Normal : Constant  Value=Ass_n4
  Sum1 : Sum  Inputs=++|
  Transpose5 : Math  Operator=transpose  SaturateOnIntegerOverflow=on
  decode : Gain  Gain=Ass_Resolution
  encode : Gain  Gain=1/Ass_Resolution
  mA2A : Gain  Gain=0.001
  AssCur : Outport
  wires:
  Product9/1 -> Transpose5/1
  ApAss/1 -> Product9/2
  Abp_PY/1 -> Product9/1
  Ss1Face1Normal/1 -> Dot Product/2
  Product1/1 -> Mux5/2
  Dot Product/1 -> Product3/2, Compare To Zero/1
  Product7/1 -> Mux5/4
  Dot Product3/1 -> Compare To Zero3/1, Product6/2
  Ss1Face3Normal/1 -> Dot Product2/2
  Ss1Face2Normal/1 -> Dot Product1/2
  Product5/1 -> Product2/2
  kS_Ass/1 -> Product3/3, Product4/3, Product6/3, Product5/3
  Dot Product1/1 -> Compare To Zero1/1, Product4/2
  Product2/1 -> Mux5/3
  Product8/1 -> Dot Product/1, Dot Product1/1, Dot Product2/1, Dot Product3/1
  Transpose5/1 -> Product8/1
  Product/1 -> Mux5/1
  Product6/1 -> Product7/2
  Dot Product2/1 -> Product5/2, Compare To Zero2/1
  Compare To Zero2/1 -> Data Type Conversion2/1
  Data Type Conversion1/1 -> Product4/1
  Sunshine/1 -> Product/1, Product1/1, Product2/1, Product7/1
  Product4/1 -> Product1/2
  Product3/1 -> Product/2
  Ss1Face4Normal/1 -> Dot Product3/2
  Compare To Zero3/1 -> Data Type Conversion3/1
  Compare To Zero/1 -> Data Type Conversion/1
  Data Type Conversion3/1 -> Product6/1
  Data Type Conversion2/1 -> Product5/1
  Data Type Conversion/1 -> Product3/1
  Sun_b/1 -> Product8/2
  Compare To Zero1/1 -> Data Type Conversion1/1
  Mux5/1 -> Sum1/2
  AssNoise/1 -> 1/ R_Ass/1
  1/ R_Ass/1 -> Sum1/1
  mA2A/1 -> AssCur/1
  Sum1/1 -> A2mA/1
  encode/1 -> Rounding Function/1
  Rounding Function/1 -> decode/1
  A2mA/1 -> encode/1
  decode/1 -> mA2A/1

== system GS_model/Subsystem2/Subsystem/Sensor/GNSS/GNSSErrModel/GNSSErrSet_Pos/GNSSErrSet_Constant ==
  R_84_in : Inport
  ErrSwitch : Inport  Port=2
  Constant : Constant
  Constant1 : Constant  Value=2
  Constant2 : Constant  Value=3
  Constant3 : Constant  Value=0
  Demux : Demux  Outputs=3
  Demux1 : Demux  Outputs=2
  Logical Operator : Logic  Operator=OR  AllPortsSameDT=off  OutDataTypeStr=boolean
  Logical Operator1 : Logic  Operator=OR  AllPortsSameDT=off  OutDataTypeStr=boolean
  Logical Operator2 : Logic  Operator=OR  AllPortsSameDT=off  OutDataTypeStr=boolean
  Memory : Memory
  Memory1 : Memory
  Memory2 : Memory
  Mux : Mux  Inputs=3
  Relational Operator{1..5,9} (6 alike) : RelationalOperator  Operator===  OutDataTypeStr=boolean  RndMeth=Simplest
  Switch1 : Switch  Criteria=u2 > Threshold  Threshold=0.5
  Switch2 : Switch  Criteria=u2 > Threshold  Threshold=0.5
  Switch3 : Switch  Criteria=u2 > Threshold  Threshold=0.5
  Triggered Subsystem1 : Subsystem  TreatAsAtomicUnit=on
  Triggered Subsystem2 : Subsystem  TreatAsAtomicUnit=on
  Triggered Subsystem8 : Subsystem  TreatAsAtomicUnit=on
  R_84_out : Outport
  wires:
  Mux/1 -> R_84_out/1
  Constant2/1 -> Relational Operator2/2
  Demux1/2 -> Triggered Subsystem1/1(In1), Triggered Subsystem2/1(In1), Triggered Subsystem8/1(In1)
  Demux1/1 -> Relational Operator4/2, Relational Operator1/1, Relational Operator5/2, Relational Operator2/1, Relational Operator3/2, Relational Operator9/1
  Constant1/1 -> Relational Operator1/2
  Triggered Subsystem8/1(Out1) -> Switch1/2
  Constant/1 -> Relational Operator9/2
  Triggered Subsystem2/1(Out1) -> Switch3/2
  Switch3/1 -> Memory2/1, Mux/3
  Memory2/1 -> Switch3/1
  Demux/3 -> Switch3/3
  Triggered Subsystem1/1(Out1) -> Switch2/2
  Switch2/1 -> Memory1/1, Mux/2
  Memory1/1 -> Switch2/1
  Demux/2 -> Switch2/3
  Demux/1 -> Switch1/3
  ErrSwitch/1 -> Demux1/1
  Memory/1 -> Switch1/1
  Switch1/1 -> Mux/1, Memory/1
  R_84_in/1 -> Demux/1
  Relational Operator9/1 -> Logical Operator/2
  Relational Operator3/1 -> Logical Operator/1
  Logical Operator/1 -> Triggered Subsystem8/Enable
  Constant3/1 -> Relational Operator5/1, Relational Operator4/1, Relational Operator3/1
  Relational Operator4/1 -> Logical Operator1/1
  Relational Operator1/1 -> Logical Operator1/2
  Logical Operator1/1 -> Triggered Subsystem1/Enable
  Relational Operator5/1 -> Logical Operator2/1
  Relational Operator2/1 -> Logical Operator2/2
  Logical Operator2/1 -> Triggered Subsystem2/Enable

== system GS_model/Subsystem2/Subsystem/Sensor/GNSS/GNSSErrModel/GNSSErrSet_Pos/GNSSErrSet_WildValue ==
  R_84_in : Inport
  ErrSwitch : Inport  Port=2
  Gain : Gain  Gain=1.5
  Switch1 : Switch  Criteria=u2 > Threshold  Threshold=0.5
  R_84_out : Outport
  wires:
  ErrSwitch/1 -> Switch1/2
  R_84_in/1 -> Switch1/3, Gain/1
  Gain/1 -> Switch1/1
  Switch1/1 -> R_84_out/1

== system GS_model/Subsystem2/Subsystem/Sensor/GNSS/GNSSErrModel/GNSSErrSet_Pos/If Action Subsystem ==
  In1 : Inport
  Action Port : ActionPort  ActionType=then
  Out1 : Outport
  wires:
  In1/1 -> Out1/1

== system GS_model/Subsystem2/Subsystem/Sensor/GNSS/GNSSErrModel/GNSSErrSet_Pos/If Action Subsystem1 ==
  In1 : Inport
  Action Port : ActionPort  ActionType=else
  Out1 : Outport
  wires:
  In1/1 -> Out1/1

== system GS_model/Subsystem2/Subsystem/Sensor/GNSS/GNSSErrModel/GNSSErrSet_Pos1/GNSSErrSet_Constant ==
  V_84_in : Inport
  ErrSwitch : Inport  Port=2
  Constant : Constant
  Constant1 : Constant  Value=2
  Constant2 : Constant  Value=3
  Constant3 : Constant  Value=0
  Demux : Demux  Outputs=3
  Demux1 : Demux  Outputs=2
  Logical Operator : Logic  Operator=OR  AllPortsSameDT=off  OutDataTypeStr=boolean
  Logical Operator1 : Logic  Operator=OR  AllPortsSameDT=off  OutDataTypeStr=boolean
  Logical Operator2 : Logic  Operator=OR  AllPortsSameDT=off  OutDataTypeStr=boolean
  Memory : Memory
  Memory1 : Memory
  Memory2 : Memory
  Mux : Mux  Inputs=3
  Relational Operator{1..5,9} (6 alike) : RelationalOperator  Operator===  OutDataTypeStr=boolean  RndMeth=Simplest
  Switch1 : Switch  Criteria=u2 > Threshold  Threshold=0.5
  Switch2 : Switch  Criteria=u2 > Threshold  Threshold=0.5
  Switch3 : Switch  Criteria=u2 > Threshold  Threshold=0.5
  Triggered Subsystem1 : Subsystem  TreatAsAtomicUnit=on
  Triggered Subsystem2 : Subsystem  TreatAsAtomicUnit=on
  Triggered Subsystem8 : Subsystem  TreatAsAtomicUnit=on
  V_84_out : Outport
  wires:
  V_84_in/1 -> Demux/1
  Switch1/1 -> Memory/1, Mux/1
  Memory/1 -> Switch1/1
  ErrSwitch/1 -> Demux1/1
  Demux/1 -> Switch1/3
  Demux/2 -> Switch2/3
  Memory1/1 -> Switch2/1
  Switch2/1 -> Mux/2, Memory1/1
  Demux/3 -> Switch3/3
  Memory2/1 -> Switch3/1
  Switch3/1 -> Mux/3, Memory2/1
  Mux/1 -> V_84_out/1
  Logical Operator2/1 -> Triggered Subsystem2/Enable
  Relational Operator2/1 -> Logical Operator2/2
  Triggered Subsystem1/1(Out1) -> Switch2/2
  Demux1/2 -> Triggered Subsystem8/1(In1), Triggered Subsystem1/1(In1), Triggered Subsystem2/1(In1)
  Relational Operator5/1 -> Logical Operator2/1
  Constant3/1 -> Relational Operator5/1, Relational Operator4/1, Relational Operator3/1
  Logical Operator1/1 -> Triggered Subsystem1/Enable
  Constant1/1 -> Relational Operator1/2
  Relational Operator1/1 -> Logical Operator1/2
  Relational Operator4/1 -> Logical Operator1/1
  Constant/1 -> Relational Operator9/2
  Triggered Subsystem8/1(Out1) -> Switch1/2
  Constant2/1 -> Relational Operator2/2
  Demux1/1 -> Relational Operator4/2, Relational Operator1/1, Relational Operator5/2, Relational Operator2/1, Relational Operator3/2, Relational Operator9/1
  Relational Operator9/1 -> Logical Operator/2
  Triggered Subsystem2/1(Out1) -> Switch3/2
  Relational Operator3/1 -> Logical Operator/1
  Logical Operator/1 -> Triggered Subsystem8/Enable

== system GS_model/Subsystem2/Subsystem/Sensor/GNSS/GNSSErrModel/GNSSErrSet_Pos1/GNSSErrSet_WildValue ==
  V_84_in : Inport
  ErrSwitch : Inport  Port=2
  Gain : Gain  Gain=1.5
  Switch1 : Switch  Criteria=u2 > Threshold  Threshold=0.5
  V_84_out : Outport
  wires:
  Switch1/1 -> V_84_out/1
  Gain/1 -> Switch1/1
  V_84_in/1 -> Gain/1, Switch1/3
  ErrSwitch/1 -> Switch1/2

== system GS_model/Subsystem2/Subsystem/Sensor/GNSS/GNSSErrModel/GNSSErrSet_Pos1/If Action Subsystem ==
  In1 : Inport
  Action Port : ActionPort  ActionType=then
  Out1 : Outport
  wires:
  In1/1 -> Out1/1

== system GS_model/Subsystem2/Subsystem/Sensor/GNSS/GNSSErrModel/GNSSErrSet_Pos1/If Action Subsystem1 ==
  In1 : Inport
  Action Port : ActionPort  ActionType=else
  Out1 : Outport
  wires:
  In1/1 -> Out1/1

== system GS_model/Subsystem2/Subsystem/Sensor/Gyro/GyroAModel/GyroErrSet/GyroErrSet ==
  Wgi : Inport
  TC_GyroErrSet_Constant : Inport  Port=2
  TC_GyroErrSet_WildValue : Inport  Port=3
  TC_GyroErrSet_Jump : Inport  Port=4
  TC_StErrSet_Wave : Inport  Port=5
  GyroErrSet_Constant : Subsystem
  GyroErrSet_Jump : Subsystem
  GyroErrSet_Wave : Subsystem
  GyroErrSet_WildValue : Subsystem
  Wgi_g : Outport
  wires:
  GyroErrSet_WildValue/1(w_out) -> GyroErrSet_Jump/1(w_in)
  GyroErrSet_Constant/1(w_out) -> GyroErrSet_WildValue/1(w_in)
  GyroErrSet_Jump/1(w_out) -> GyroErrSet_Wave/1(w_in)
  Wgi/1 -> GyroErrSet_Constant/1(w_in)
  TC_GyroErrSet_Constant/1 -> GyroErrSet_Constant/2(ErrSwitch)
  TC_GyroErrSet_WildValue/1 -> GyroErrSet_WildValue/2(ErrSwitch)
  TC_GyroErrSet_Jump/1 -> GyroErrSet_Jump/2(ErrSet)
  TC_StErrSet_Wave/1 -> GyroErrSet_Wave/2(ErrSet)
  GyroErrSet_Wave/1(w_out) -> Wgi_g/1

== system GS_model/Subsystem2/Subsystem/Sensor/Gyro/GyroAModel/GyroErrSet/If Action Subsystem3 ==
  In1 : Inport
  Action Port : ActionPort  ActionType=else
  Out1 : Outport
  wires:
  In1/1 -> Out1/1

== system GS_model/Subsystem2/Subsystem/Sensor/Gyro/GyroAModel/GyroErrSet/If Action Subsystem4 ==
  In1 : Inport
  Action Port : ActionPort  ActionType=then
  Gain : Gain  Gain=DEG2RAD
  Out1 : Outport
  wires:
  In1/1 -> Gain/1
  Gain/1 -> Out1/1

== system GS_model/Subsystem2/Subsystem/Sensor/Gyro/GyroAModel/GyroErrSet/Triggered Subsystem5 ==
  In1 : Inport
  Enable : EnablePort
  Out1 : Outport  InitialOutput=0
  wires:
  In1/1 -> Out1/1

== system GS_model/Subsystem2/Subsystem/Sensor/Gyro/GyroAModel/GyroErrSet/Triggered Subsystem6 ==
  In1 : Inport
  Enable : EnablePort
  Out1 : Outport  InitialOutput=0
  wires:
  In1/1 -> Out1/1

== system GS_model/Subsystem2/Subsystem/Sensor/Gyro/GyroAModel/GyroErrSet/Triggered Subsystem7 ==
  In1 : Inport
  Enable : EnablePort
  Out1 : Outport
  wires:
  In1/1 -> Out1/1

== system GS_model/Subsystem2/Subsystem/Sensor/Gyro/GyroAModel/GyroErrSet/Triggered Subsystem8 ==
  In1 : Inport
  Enable : EnablePort
  Out1 : Outport
  wires:
  In1/1 -> Out1/1

== system GS_model/Subsystem2/Subsystem/Sensor/Gyro/GyroAModel/GyroErrSet/Triggered Subsystem9 ==
  In1 : Inport
  Enable : EnablePort
  Out1 : Outport
  wires:
  In1/1 -> Out1/1

== system GS_model/Subsystem2/Subsystem/Sensor/Gyro/GyroAModel/GyroMathModel/Triggered Subsystem1 ==
  In1 : Inport
  Enable : EnablePort
  Out1 : Outport  InitialOutput=0
  wires:
  In1/1 -> Out1/1
